simulink model "M46D"  (R2015a)
settings: Solver=ode45  StartTime=0.0  StopTime=20.0  RelTol=1e-4
values from neighbouring files (symbols this model uses):
  d1 = 500    [DePascali4Minit.m]    (also in M46Dinit.m)
  d2 = 500    [DePascali4Minit.m]    (also in M46Dinit.m)
  d3 = 500    [DePascali4Minit.m]    (also in M46Dinit.m)
  d4 = 500    [DePascali4Minit.m]    (also in M46Dinit.m)
  delta1 = 200    [DePascali4Minit.m]    (also in M46Dinit.m)
  delta2 = 200    [DePascali4Minit.m]    (also in M46Dinit.m)
  delta3 = 200    [DePascali4Minit.m]    (also in M46Dinit.m)
  delta4 = 200    [DePascali4Minit.m]    (also in M46Dinit.m)
  g = [0;0;9.81]    [DePascali4Minit.m]    (also in M46Dinit.m)
  j0 = 0.5    [DePascali4Minit.m]    (also in M46Dinit.m)
  j1 = 10    [DePascali4Minit.m]    (also in M46Dinit.m = 1)
  j2 = 10    [DePascali4Minit.m]    (also in M46Dinit.m = 1)
  j3 = 10    [DePascali4Minit.m]    (also in M46Dinit.m = 1)
  j4 = 10    [DePascali4Minit.m]    (also in M46Dinit.m = 1)
  k1 = 50    [DePascali4Minit.m]    (also in M46Dinit.m = 100)
  k2 = 50    [DePascali4Minit.m]    (also in M46Dinit.m = 100)
  k3 = 50    [DePascali4Minit.m]    (also in M46Dinit.m = 100)
  k4 = 50    [DePascali4Minit.m]    (also in M46Dinit.m = 100)
  kappa1 = 10    [DePascali4Minit.m]    (also in M46Dinit.m = 100)
  kappa2 = 10    [DePascali4Minit.m]    (also in M46Dinit.m = 100)
  kappa3 = 10    [DePascali4Minit.m]    (also in M46Dinit.m = 100)
  kappa4 = 10    [DePascali4Minit.m]    (also in M46Dinit.m = 100)
  m0 = 20    [DePascali4Minit.m]    (also in M46Dinit.m)
  m1 = 100    [DePascali4Minit.m]    (also in M46Dinit.m = 10)
  m2 = 100    [DePascali4Minit.m]    (also in M46Dinit.m = 10)
  m3 = 100    [DePascali4Minit.m]    (also in M46Dinit.m = 10)
  m4 = 100    [DePascali4Minit.m]    (also in M46Dinit.m = 10)
  r = [1; 0; 0 ... (first row only)    [DePascali4Minit.m]    (also in M46Dinit.m)
undefined symbols (not defined in the file or in its folder): A, G_Mplus
libraries: aerolibutil x10, aerolibtransform2 x8, dspinverses x3
settings Model: CovSFcnEnable=off  Creator=Martin  LastModifiedBy=mangerer
settings DebuggingCC: SolverPrmCheckMsg=warning

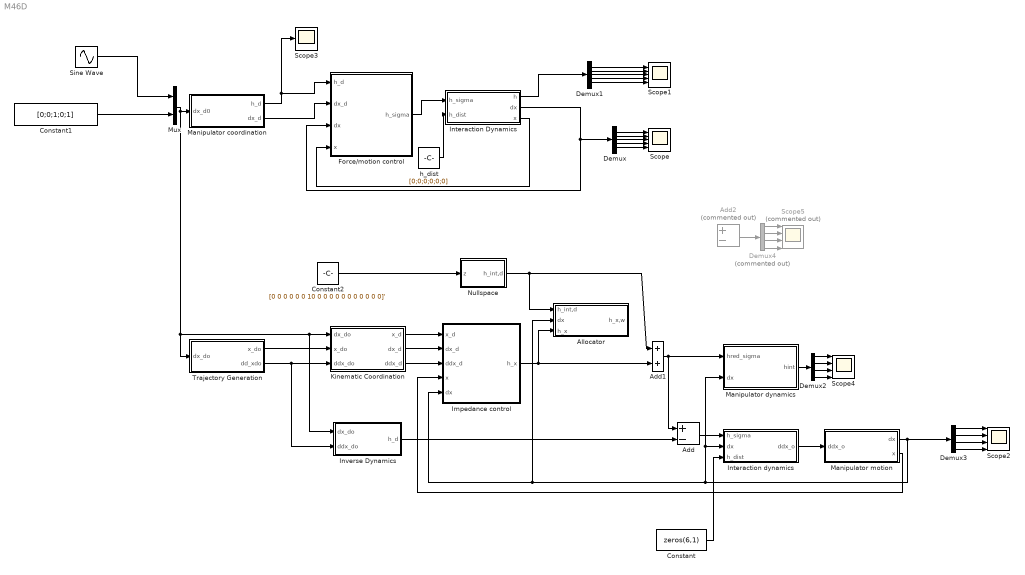
== system M46D ==
  Add : Sum  Inputs=+-
  Add1 : Sum
  Add2 : Sum  Commented=on  Inputs=+-
  Allocator : Subsystem
  Constant : Constant  Value=zeros(6,1)
  Constant1 : Constant  Value=[0;0;1;0;1]
  Constant2 : Constant  Value=[0 0 0 0 0 0 10 0 0 0 0 0 0 0 0 0 0 0]'
  Demux : Demux  Outputs=5
  Demux1 : Demux  Outputs=5
  Demux2 : Demux
  Demux3 : Demux
  Demux4 : Demux  Commented=on
  Force/motion control : Subsystem
  Impedance control : Subsystem
  Interaction Dynamics : Subsystem
  Interaction dynamics : Subsystem
  Inverse Dynamics : Subsystem
  Kinematic Coordination : Subsystem
  Manipulator coordination : Subsystem
  Manipulator dynamics : Subsystem
  Manipulator motion : Subsystem
  Mux : Mux  Inputs=2
  Nullspace : Subsystem
  Scope : Scope  NumInputPorts=5
      settings: ShowLegends=on  YMin=-1.25~-1.25~-2.5~-1.25~-1.5  YMax=1.25~1.25~1.5~1.25~2
  Scope1 : Scope  NumInputPorts=5
      settings: ShowLegends=on  YMin=-50~-100~-100~-5~-5  YMax=200~20~20~5~5
  Scope2 : Scope  NumInputPorts=4
      settings: ShowLegends=on  YMin=-1.25~-2.25~-1.25~-1  YMax=1.25~1.25~1.25~2.25  SaveName=ScopeData2
  Scope3 : Scope
      settings: SaveName=ScopeData5
  Scope4 : Scope  NumInputPorts=4
      settings: ShowLegends=on  YMin=-25~-12.5~-20~-12.5  YMax=20~10~25~7.5  SaveName=ScopeData8
  Scope5 : Scope  Commented=on  NumInputPorts=4
      settings: ShowLegends=on  YMin=-3~-0.5~-0.5~-2.5  YMax=5~2.5~2.5~0.5  SaveName=ScopeData10
  Sine Wave : Sin  SampleTime=0
  Trajectory Generation : Subsystem
  h_dist : Constant  Value=[0;0;0;0;0;0]
  wires:
  Interaction Dynamics/2(dx) -> Force/motion control/3(dx), Demux/1
  Demux/1 -> Scope/1
  Demux/2 -> Scope/2
  Demux/3 -> Scope/3
  Force/motion control/1(h_sigma) -> Interaction Dynamics/1(h_sigma)
  Manipulator coordination/2(dx_d) -> Force/motion control/2(dx_d)
  Interaction Dynamics/1(h) -> Demux1/1
  Demux1/1 -> Scope1/1
  Demux1/2 -> Scope1/2
  Demux1/3 -> Scope1/3
  h_dist/1 -> Interaction Dynamics/2(h_dist)
  Manipulator coordination/1(h_d) -> Force/motion control/1(h_d), Scope3/1
  Mux/1 -> Inverse Dynamics/1(dx_do), Kinematic Coordination/1(dx_do), Trajectory Generation/1(dx_do), Manipulator coordination/1(dx_d0)
  Interaction Dynamics/3(x) -> Force/motion control/4(x)
  Demux1/4 -> Scope1/4
  Demux1/5 -> Scope1/5
  Demux/4 -> Scope/4
  Demux/5 -> Scope/5
  Trajectory Generation/1(x_do) -> Kinematic Coordination/2(x_do)
  Trajectory Generation/2(dd_xdo) -> Inverse Dynamics/2(ddx_do), Kinematic Coordination/3(ddx_do)
  Kinematic Coordination/1(x_d) -> Impedance control/1(x_d)
  Kinematic Coordination/2(dx_d) -> Impedance control/2(dx_d)
  Kinematic Coordination/3(ddx_d) -> Impedance control/3(ddx_d)
  Interaction dynamics/1(ddx_o) -> Manipulator motion/1(ddx_o)
  Impedance control/1(h_x) -> Add1/2, Allocator/3(h_x)
  Inverse Dynamics/1(h_d) -> Add/2
  Add/1 -> Interaction dynamics/1(h_sigma)
  Manipulator motion/1(dx) -> Demux3/1, Allocator/2(dx), Impedance control/5(dx), Interaction dynamics/2(dx), Manipulator dynamics/2(dx)
  Manipulator motion/2(x) -> Impedance control/4(x)
  Constant/1 -> Interaction dynamics/3(h_dist)
  Manipulator dynamics/1(hint) -> Demux2/1
  Demux2/1 -> Scope4/1
  Demux2/2 -> Scope4/2
  Demux2/3 -> Scope4/3
  Demux2/4 -> Scope4/4
  Constant1/1 -> Mux/2
  Sine Wave/1 -> Mux/1
  Demux3/1 -> Scope2/1
  Demux3/2 -> Scope2/2
  Demux3/3 -> Scope2/3
  Demux3/4 -> Scope2/4
  Add1/1 -> Add/1, Manipulator dynamics/1(hred_sigma)
  Constant2/1 -> Nullspace/1(z)
  Demux4/1 -> Scope5/1
  Demux4/2 -> Scope5/2
  Demux4/3 -> Scope5/3
  Demux4/4 -> Scope5/4
  Add2/1 -> Demux4/1
  Nullspace/1(h_int,d) -> Allocator/1(h_int,d), Add1/1

== system M46D/Allocator ==
  h_int,d : Inport
  dx : Inport  Port=2
  h_x : Inport  Port=3
  Add : Sum  Inputs=-+
  Add1 : Sum
  Divide : Product  Inputs=*/*  Multiplication=Matrix(*)
  Divide1 : Product  Inputs=*/*  Multiplication=Matrix(*)
  Divide2 : Product  Inputs=*/*  Multiplication=Matrix(*)
  Inertia : Constant  Value=blkdiag(m1*eye(3), j1*eye(3), m2*eye(3), j2*eye(3), m3*eye(3), j3*eye(3), m4*eye(3), j3*eye(3))
  MATLAB Function : MATLAB Function  TreatAsAtomicUnit=on
  MATLAB Function1 : MATLAB Function  TreatAsAtomicUnit=on
  Math Function : Math  Operator=transpose  SaturateOnIntegerOverflow=on
  h_x,w : Outport
  wires:
  dx/1 -> MATLAB Function1/1(dx)
  Divide/1 -> h_x,w/1
  Math Function/1 -> Divide1/3, Divide/1
  MATLAB Function/1(Ared) -> Math Function/1, Divide2/1, Divide1/1
  Divide1/1 -> Divide/2
  Inertia/1 -> Divide1/2, Divide2/2
  MATLAB Function1/1(bred) -> Add/2
  Add/1 -> Divide/3
  Divide2/1 -> Add/1
  Add1/1 -> Divide2/3
  h_int,d/1 -> Add1/1
  h_x/1 -> Add1/2

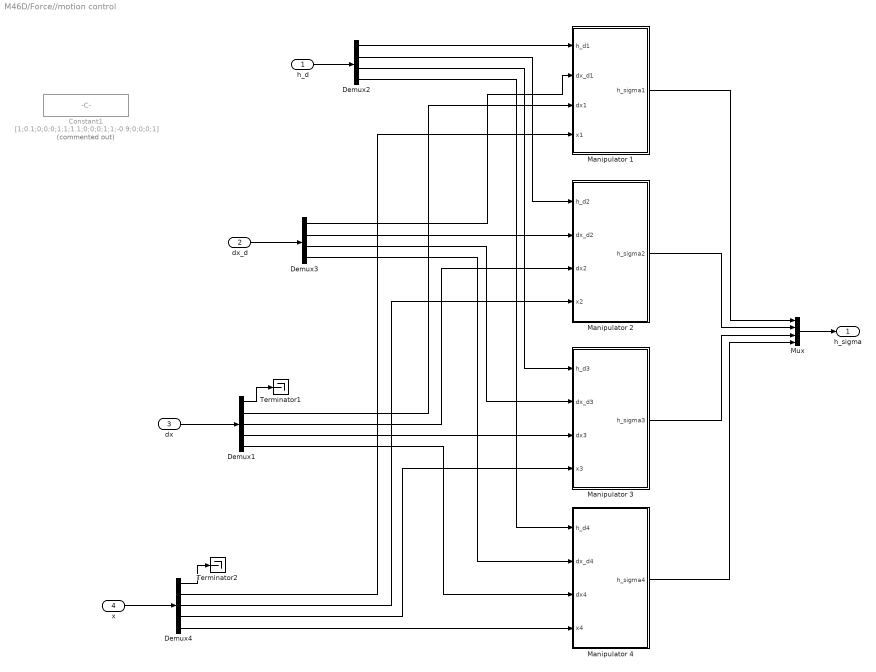
== system M46D/Force//motion control ==
  h_d : Inport
  dx_d : Inport  Port=2
  dx : Inport  Port=3
  x : Inport  Port=4
  Constant1 : Constant  Commented=on  Value=[1;0.1;0;0;0;1;1;1.1;0;0;0;1;1;-0.9;0;0;0;1]
  Demux1 : Demux  Outputs=5
  Demux2 : Demux
  Demux3 : Demux
  Demux4 : Demux  Outputs=5
  Manipulator 1 : Subsystem
  Manipulator 2 : Subsystem
  Manipulator 3 : Subsystem
  Manipulator 4 : Subsystem
  Mux : Mux
  Terminator1 : Terminator
  Terminator2 : Terminator
  h_sigma : Outport
  wires:
  Manipulator 1/1(h_sigma1) -> Mux/1
  Manipulator 2/1(h_sigma2) -> Mux/2
  Mux/1 -> h_sigma/1
  Demux1/1 -> Terminator1/1
  dx_d/1 -> Demux3/1
  h_d/1 -> Demux2/1
  dx/1 -> Demux1/1
  x/1 -> Demux4/1
  Demux4/1 -> Terminator2/1
  Manipulator 3/1(h_sigma3) -> Mux/3
  Manipulator 4/1(h_sigma4) -> Mux/4
  Demux4/5 -> Manipulator 4/4(x4)
  Demux2/1 -> Manipulator 1/1(h_d1)
  Demux2/2 -> Manipulator 2/1(h_d2)
  Demux2/3 -> Manipulator 3/1(h_d3)
  Demux2/4 -> Manipulator 4/1(h_d4)
  Demux3/1 -> Manipulator 1/2(dx_d1)
  Demux3/2 -> Manipulator 2/2(dx_d2)
  Demux3/3 -> Manipulator 3/2(dx_d3)
  Demux3/4 -> Manipulator 4/2(dx_d4)
  Demux1/2 -> Manipulator 1/3(dx1)
  Demux1/3 -> Manipulator 2/3(dx2)
  Demux1/4 -> Manipulator 3/3(dx3)
  Demux1/5 -> Manipulator 4/3(dx4)
  Demux4/4 -> Manipulator 3/4(x3)
  Demux4/3 -> Manipulator 2/4(x2)
  Demux4/2 -> Manipulator 1/4(x1)

== system M46D/Impedance control ==
  x_d : Inport
  dx_d : Inport  Port=2
  ddx_d : Inport  Port=3
  x : Inport  Port=4
  dx : Inport  Port=5
  Demux{,1..4} (5 alike) : Demux
  Manipulator1 : Subsystem
  Manipulator2 : Subsystem
  Manipulator3 : Subsystem
  Manipulator4 : Subsystem
  Mux : Mux
  h_x : Outport
  wires:
  dx/1 -> Demux4/1
  x/1 -> Demux3/1
  ddx_d/1 -> Demux2/1
  dx_d/1 -> Demux1/1
  x_d/1 -> Demux/1
  Demux/1 -> Manipulator1/1(x_d1)
  Demux/2 -> Manipulator2/1(x_d2)
  Demux/3 -> Manipulator3/1(x_d3)
  Demux/4 -> Manipulator4/1(x_d4)
  Demux1/1 -> Manipulator1/2(dx_d1)
  Demux1/2 -> Manipulator2/2(dx_d2)
  Demux1/3 -> Manipulator3/2(dx_d3)
  Demux1/4 -> Manipulator4/2(dx_d4)
  Demux2/1 -> Manipulator1/3(ddx_d1)
  Demux2/2 -> Manipulator2/3(ddx_d2)
  Demux2/3 -> Manipulator3/3(ddx_d3)
  Demux2/4 -> Manipulator4/3(ddx_d4)
  Demux3/1 -> Manipulator1/4(x1)
  Demux3/2 -> Manipulator2/4(x2)
  Demux3/3 -> Manipulator3/4(x3)
  Demux3/4 -> Manipulator4/4(x4)
  Demux4/4 -> Manipulator4/5(dx4)
  Demux4/3 -> Manipulator3/5(dx3)
  Demux4/2 -> Manipulator2/5(dx2)
  Demux4/1 -> Manipulator1/5(dx1)
  Mux/1 -> h_x/1
  Manipulator1/1(h_x1) -> Mux/1
  Manipulator2/1(h_x2) -> Mux/2
  Manipulator3/1(h_x3) -> Mux/3
  Manipulator4/1(h_x4) -> Mux/4

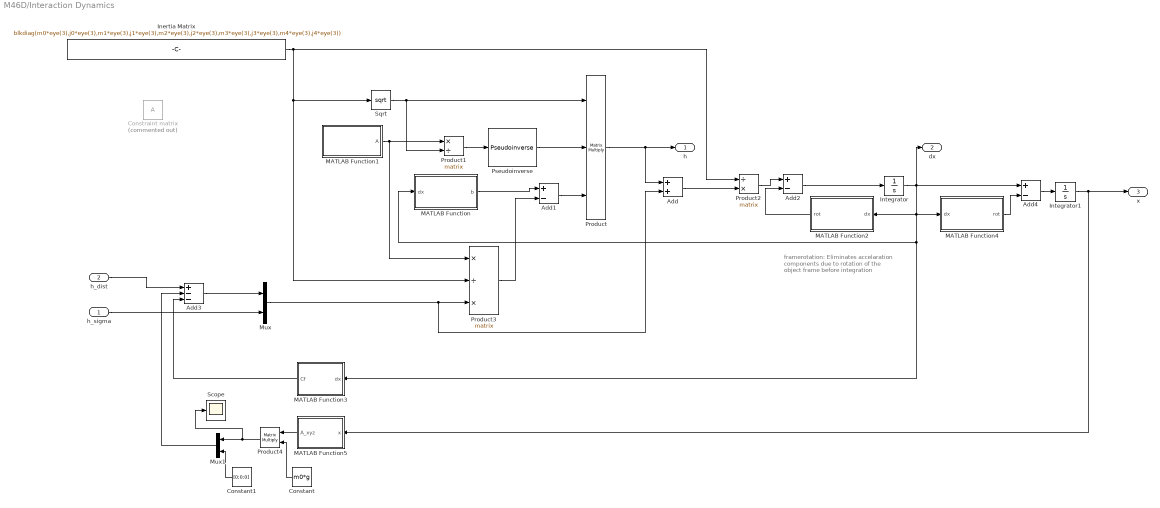
== system M46D/Interaction Dynamics ==
  note: framerotation: Eliminates accelaration
      |  components  due to rotation of the
      |  object frame before integration
  h_sigma : Inport
  h_dist : Inport  Port=2
  Add : Sum
  Add1 : Sum  Inputs=+-
  Add2 : Sum  Inputs=+-
  Add3 : Sum  Inputs=+--
  Add4 : Sum  Inputs=+-
  Constant : Constant  Value=m0*g
  Constant1 : Constant  Value=[0;0;0]
  Constraint matrix : Constant  Commented=on  Value=A
  Inertia Matrix : Constant  Value=blkdiag(m0*eye(3),j0*eye(3),m1*eye(3),j1*eye(3),m2*eye(3),j2*eye(3),m3*eye(3),j3*eye(3),m4*eye(3),j4*eye(3))
  Integrator : Integrator
  Integrator1 : Integrator
  MATLAB Function : MATLAB Function  TreatAsAtomicUnit=on
  MATLAB Function1 : MATLAB Function  TreatAsAtomicUnit=on
  MATLAB Function2 : MATLAB Function  TreatAsAtomicUnit=on
  MATLAB Function3 : MATLAB Function  TreatAsAtomicUnit=on
  MATLAB Function4 : MATLAB Function  TreatAsAtomicUnit=on
  MATLAB Function5 : MATLAB Function  TreatAsAtomicUnit=on
  Mux : Mux  Inputs=2
  Mux1 : Mux  Inputs=2
  Product : Product  Inputs=***  Multiplication=Matrix(*)
  Product1 : Product  Inputs=*/  Multiplication=Matrix(*)
  Product2 : Product  Inputs=/*  Multiplication=Matrix(*)
  Product3 : Product  Inputs=*/*  Multiplication=Matrix(*)
  Product4 : Product  Multiplication=Matrix(*)
  Pseudoinverse : dspinverses/Pseudoinverse  wanterr=off
  Scope : Scope
      settings: ShowLegends=on  SaveName=ScopeData6
  Sqrt : Sqrt  SaturateOnIntegerOverflow=on
  h : Outport
  dx : Outport  Port=2
  x : Outport  Port=3
  wires:
  Sqrt/1 -> Product/1, Product1/2
  Pseudoinverse/1 -> Product/2
  Product1/1 -> Pseudoinverse/1
  Integrator/1 -> dx/1, Add4/1, MATLAB Function4/1(dx), MATLAB Function2/1(dx), MATLAB Function3/1(dx), MATLAB Function/1(dx)
  Product/1 -> h/1, Add/1
  Add/1 -> Product2/2
  Inertia Matrix/1 -> Product2/1, Sqrt/1, Product3/2
  h_sigma/1 -> Mux/2
  Add1/1 -> Product/3
  MATLAB Function/1(b) -> Add1/1
  Product3/1 -> Add1/2
  Mux/1 -> Add/2, Product3/3
  MATLAB Function1/1(A) -> Product1/1, Product3/1
  Product2/1 -> Add2/1
  Add2/1 -> Integrator/1
  MATLAB Function2/1(rot) -> Add2/2
  Add3/1 -> Mux/1
  h_dist/1 -> Add3/1
  Integrator1/1 -> MATLAB Function5/1(x), x/1
  Add4/1 -> Integrator1/1
  MATLAB Function4/1(rot) -> Add4/2
  MATLAB Function5/1(A_xyz) -> Product4/1
  MATLAB Function3/1(Cf) -> Add3/3
  Constant/1 -> Product4/2
  Product4/1 -> Scope/1, Mux1/1
  Constant1/1 -> Mux1/2
  Mux1/1 -> Add3/2

== system M46D/Interaction dynamics ==
  h_sigma : Inport
  dx : Inport  Port=2
  h_dist : Inport  Port=3
  Add : Sum  Inputs=++-
  Add1 : Sum  Inputs=+--
  Gravitation : Constant  Value=[-m0*g;zeros(3,1)]
  Inertia : Constant  Value=blkdiag(m1*eye(3), j1*eye(3), m2*eye(3), j2*eye(3), m3*eye(3), j3*eye(3), m4*eye(3), j3*eye(3))
  MATLAB Function : MATLAB Function  TreatAsAtomicUnit=on
  MATLAB Function1 : MATLAB Function  TreatAsAtomicUnit=on
  MATLAB Function2 : MATLAB Function  TreatAsAtomicUnit=on
  MATLAB Function3 : MATLAB Function  TreatAsAtomicUnit=on
  Product : Product  Inputs=/*  Multiplication=Matrix(*)
  Product1 : Product  Multiplication=Matrix(*)
  Product3 : Product  Inputs=***  Multiplication=Matrix(*)
  ddx_o : Outport
  wires:
  MATLAB Function3/1(G) -> Product1/1, Product3/1, MATLAB Function/1(G)
  Inertia/1 -> Product3/2, MATLAB Function/2(M)
  MATLAB Function/1(Mapp) -> Product/1
  Add/1 -> Product/2
  Product1/1 -> Add/2
  h_sigma/1 -> Product1/2
  Add1/1 -> Add/1
  h_dist/1 -> Add1/1
  Gravitation/1 -> Add1/2
  dx/1 -> MATLAB Function2/1(dx), MATLAB Function1/1(dx)
  MATLAB Function1/1(hcoriolis) -> Add1/3
  Product3/1 -> Add/3
  MATLAB Function2/1(b) -> Product3/3
  Product/1 -> ddx_o/1

== system M46D/Inverse Dynamics ==
  dx_do : Inport
  ddx_do : Inport  Port=2
  Add : Sum  Inputs=+++
  Gravitation : Constant  Value=[-m0*g;zeros(3,1)]
  MATLAB Function : MATLAB Function  TreatAsAtomicUnit=on
  MATLAB Function3 : MATLAB Function  TreatAsAtomicUnit=on
  Object Inertia : Constant  Value=blkdiag(m0*eye(3),j0*eye(3));
  Product : Product  Multiplication=Matrix(*)
  Product1 : Product  Multiplication=Matrix(*)
  Product2 : Product  Multiplication=Matrix(*)
  Pseudoinverse : dspinverses/Pseudoinverse  wanterr=off
  h_d : Outport
  wires:
  ddx_do/1 -> Product/2
  Object Inertia/1 -> Product/1
  Product/1 -> Add/3
  dx_do/1 -> Product1/2, MATLAB Function/1(dx_do)
  MATLAB Function/1(C_o) -> Product1/1
  Product1/1 -> Add/2
  Gravitation/1 -> Add/1
  MATLAB Function3/1(G) -> Pseudoinverse/1
  Add/1 -> Product2/2
  Pseudoinverse/1 -> Product2/1
  Product2/1 -> h_d/1

== system M46D/Kinematic Coordination ==
  dx_do : Inport
  x_do : Inport  Port=2
  ddx_do : Inport  Port=3
  Add : Sum
  Demux : Demux  Outputs=7
  MATLAB Function : MATLAB Function  TreatAsAtomicUnit=on
  MATLAB Function1 : MATLAB Function  TreatAsAtomicUnit=on
  MATLAB Function3 : MATLAB Function  TreatAsAtomicUnit=on
  Math Function : Math  Operator=transpose  SaturateOnIntegerOverflow=on
  Mux : Mux  Inputs=3
  Mux1 : Mux
  Product : Product  Multiplication=Matrix(*)
  Product1 : Product  Multiplication=Matrix(*)
  x_d : Outport
  dx_d : Outport  Port=2
  ddx_d : Outport  Port=3
  wires:
  MATLAB Function3/1(G) -> Math Function/1
  Math Function/1 -> Product1/1, Product/1
  dx_do/1 -> MATLAB Function1/1(dx_do), Product/2
  Product/1 -> dx_d/1
  x_do/1 -> Demux/1
  Demux/1 -> Mux/1
  Demux/2 -> Mux/2
  Demux/3 -> Mux/3
  Demux/5 -> Mux1/2
  Demux/6 -> Mux1/3
  Demux/7 -> Mux1/4
  Demux/4 -> Mux1/1
  Mux1/1 -> MATLAB Function/2(q_do)
  Mux/1 -> MATLAB Function/1(p_do)
  MATLAB Function/1(x_d) -> x_d/1
  MATLAB Function1/1(b) -> Add/1
  ddx_do/1 -> Product1/2
  Product1/1 -> Add/2
  Add/1 -> ddx_d/1

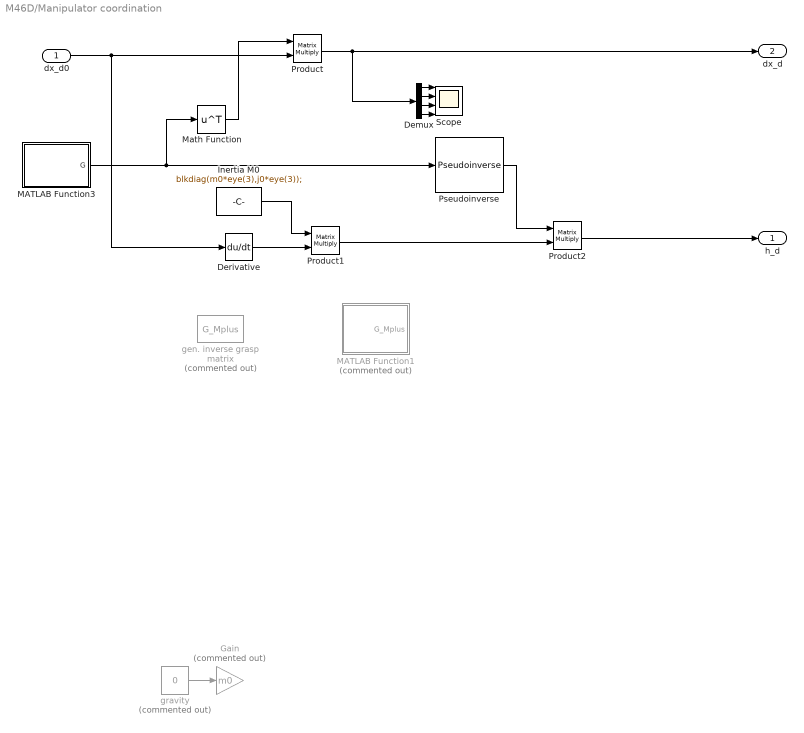
== system M46D/Manipulator coordination ==
  dx_d0 : Inport
  Demux : Demux
  Derivative : Derivative
  Gain : Gain  Commented=on  Gain=m0
  Inertia M0 : Constant  Value=blkdiag(m0*eye(3),j0*eye(3));
  MATLAB Function1 : MATLAB Function  Commented=on  TreatAsAtomicUnit=on
  MATLAB Function3 : MATLAB Function  TreatAsAtomicUnit=on
  Math Function : Math  Operator=transpose  SaturateOnIntegerOverflow=on
  Product : Product  Multiplication=Matrix(*)
  Product1 : Product  Multiplication=Matrix(*)
  Product2 : Product  Multiplication=Matrix(*)
  Pseudoinverse : dspinverses/Pseudoinverse  wanterr=off
  Scope : Scope  NumInputPorts=4
      settings: ShowLegends=on  YMin=-5~-5~-5~-5  YMax=5~5~5~5  SaveName=ScopeData3
  gen. inverse grasp matrix : Constant  Commented=on  Value=G_Mplus
  gravity : Constant  Commented=on  Value=0
  h_d : Outport
  dx_d : Outport  Port=2
  wires:
  dx_d0/1 -> Product/2, Derivative/1
  Math Function/1 -> Product/1
  Product/1 -> Demux/1, dx_d/1
  Derivative/1 -> Product1/2
  gravity/1 -> Gain/1
  Product1/1 -> Product2/2
  Product2/1 -> h_d/1
  Demux/1 -> Scope/1
  Demux/2 -> Scope/2
  Demux/3 -> Scope/3
  Demux/4 -> Scope/4
  Inertia M0/1 -> Product1/1
  MATLAB Function3/1(G) -> Pseudoinverse/1, Math Function/1
  Pseudoinverse/1 -> Product2/1

== system M46D/Manipulator dynamics ==
  hred_sigma : Inport
  dx : Inport  Port=2
  Add : Sum  Inputs=-+
  Divide : Product  Inputs=*/*  Multiplication=Matrix(*)
  Divide1 : Product  Inputs=*/*  Multiplication=Matrix(*)
  Divide2 : Product  Inputs=*/*  Multiplication=Matrix(*)
  Inertia : Constant  Value=blkdiag(m1*eye(3), j1*eye(3), m2*eye(3), j2*eye(3), m3*eye(3), j3*eye(3), m4*eye(3), j3*eye(3))
  MATLAB Function : MATLAB Function  TreatAsAtomicUnit=on
  MATLAB Function1 : MATLAB Function  TreatAsAtomicUnit=on
  Math Function : Math  Operator=transpose  SaturateOnIntegerOverflow=on
  hint : Outport
  wires:
  Divide/1 -> hint/1
  Math Function/1 -> Divide1/3, Divide/1
  MATLAB Function/1(Ared) -> Math Function/1, Divide2/1, Divide1/1
  Divide1/1 -> Divide/2
  Inertia/1 -> Divide1/2, Divide2/2
  dx/1 -> MATLAB Function1/1(dx)
  MATLAB Function1/1(bred) -> Add/2
  Add/1 -> Divide/3
  Divide2/1 -> Add/1
  hred_sigma/1 -> Divide2/3

== system M46D/Manipulator motion ==
  ddx_o : Inport
  AngVelo2Quat : Subsystem
  Demux : Demux  Outputs=2
  Integrator : Integrator  InitialCondition=zeros(6,1)
  Integrator1 : Integrator  InitialCondition=[0 0 0]'
  MATLAB Function : MATLAB Function  TreatAsAtomicUnit=on
  MATLAB Function3 : MATLAB Function  TreatAsAtomicUnit=on
  Math Function : Math  Operator=transpose  SaturateOnIntegerOverflow=on
  Product : Product  Multiplication=Matrix(*)
  dx : Outport
  x : Outport  Port=2
  wires:
  ddx_o/1 -> Integrator/1
  Integrator/1 -> Product/2, Demux/1
  MATLAB Function3/1(G) -> Math Function/1
  Math Function/1 -> Product/1
  Product/1 -> dx/1
  Demux/2 -> AngVelo2Quat/1(omega_o)
  Demux/1 -> Integrator1/1
  AngVelo2Quat/1(q_o) -> MATLAB Function/2(q_o)
  Integrator1/1 -> MATLAB Function/1(p_o)
  MATLAB Function/1(x) -> x/1

== system M46D/Nullspace ==
  z : Inport
  MATLAB Function : MATLAB Function  TreatAsAtomicUnit=on
  Math Function : Math  Operator=transpose  SaturateOnIntegerOverflow=on
  Product : Product  Multiplication=Matrix(*)
  h_int,d : Outport
  wires:
  MATLAB Function/1(Ared) -> Math Function/1
  Math Function/1 -> Product/1
  z/1 -> Product/2
  Product/1 -> h_int,d/1

== system M46D/Trajectory Generation ==
  dx_do : Inport
  AngVelo2Quat : Subsystem
  Demux : Demux  Outputs=2
  Derivative : Derivative
  Integrator : Integrator
  Mux : Mux  Inputs=2
  x_do : Outport
  dd_xdo : Outport  Port=2
  wires:
  dx_do/1 -> Derivative/1, Demux/1
  Demux/2 -> AngVelo2Quat/1(omega_do)
  Demux/1 -> Integrator/1
  AngVelo2Quat/1(q_do) -> Mux/2
  Integrator/1 -> Mux/1
  Mux/1 -> x_do/1
  Derivative/1 -> dd_xdo/1

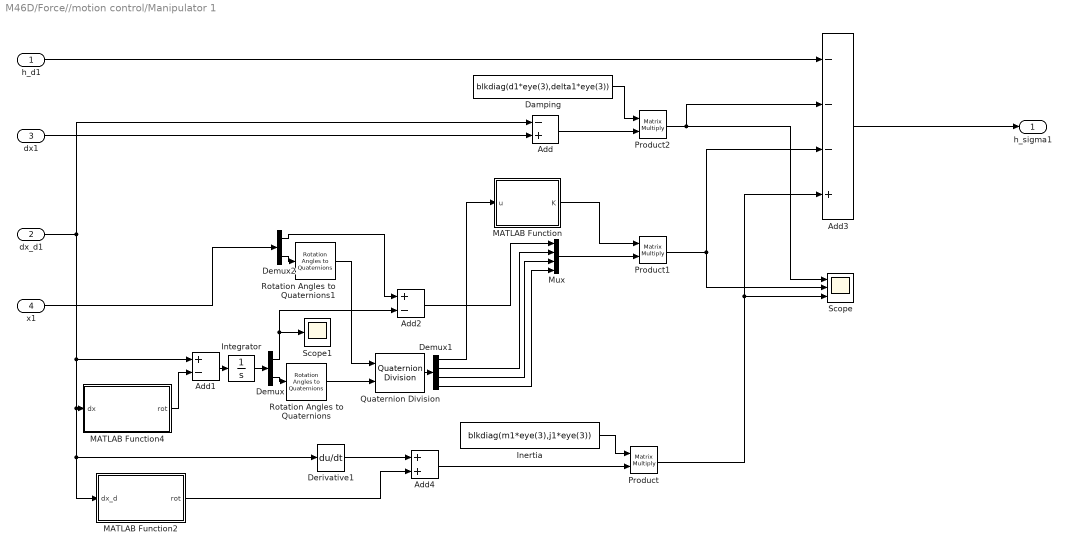
== system M46D/Force//motion control/Manipulator 1 ==
  h_d1 : Inport
  dx_d1 : Inport  Port=2
  dx1 : Inport  Port=3
  x1 : Inport  Port=4
  Add : Sum  Inputs=-+
  Add1 : Sum  Inputs=+-
  Add2 : Sum  Inputs=+-
  Add3 : Sum  Inputs=---+
  Add4 : Sum
  Damping : Constant  Value=blkdiag(d1*eye(3),delta1*eye(3))
  Demux : Demux  Outputs=2
  Demux1 : Demux
  Demux2 : Demux  Outputs=2
  Derivative1 : Derivative
  Inertia : Constant  Value=blkdiag(m1*eye(3),j1*eye(3))
  Integrator : Integrator
  MATLAB Function : MATLAB Function  TreatAsAtomicUnit=on
  MATLAB Function2 : MATLAB Function  TreatAsAtomicUnit=on
  MATLAB Function4 : MATLAB Function  TreatAsAtomicUnit=on
  Mux : Mux
  Product : Product  Multiplication=Matrix(*)
  Product1 : Product  Multiplication=Matrix(*)
  Product2 : Product  Multiplication=Matrix(*)
  Quaternion Division : aerolibutil/Quaternion Division
  Rotation Angles to Quaternions : aerolibtransform2/Rotation Angles to Quaternions  rotationOrder=XYZ
  Rotation Angles to Quaternions1 : aerolibtransform2/Rotation Angles to Quaternions  rotationOrder=XYZ
  Scope : Scope  NumInputPorts=3
      settings: ShowLegends=on  YMin=-5~-5~-5  YMax=5~5~5  SaveName=ScopeData4
  Scope1 : Scope
      settings: ShowLegends=on  SaveName=ScopeData7
  h_sigma1 : Outport
  wires:
  dx_d1/1 -> Add1/1, Derivative1/1, MATLAB Function2/1(dx_d), MATLAB Function4/1(dx), Add/1
  Mux/1 -> Product1/2
  Add/1 -> Product2/2
  Damping/1 -> Product2/1
  Inertia/1 -> Product/1
  Product/1 -> Scope/3, Add3/4
  h_d1/1 -> Add3/1
  Add3/1 -> h_sigma1/1
  Integrator/1 -> Demux/1
  Demux/2 -> Rotation Angles to Quaternions/1
  dx1/1 -> Add/2
  x1/1 -> Demux2/1
  Demux2/2 -> Rotation Angles to Quaternions1/1
  MATLAB Function/1(K) -> Product1/1
  Rotation Angles to Quaternions1/1 -> Quaternion Division/1
  Rotation Angles to Quaternions/1 -> Quaternion Division/2
  Quaternion Division/1 -> Demux1/1
  Demux1/1 -> MATLAB Function/1(u)
  Demux2/1 -> Add2/1
  Demux/1 -> Scope1/1, Add2/2
  Add2/1 -> Mux/1
  Demux1/2 -> Mux/2
  Demux1/3 -> Mux/3
  Demux1/4 -> Mux/4
  Product2/1 -> Scope/1, Add3/2
  Product1/1 -> Add3/3, Scope/2
  MATLAB Function4/1(rot) -> Add1/2
  Add1/1 -> Integrator/1
  Add4/1 -> Product/2
  Derivative1/1 -> Add4/1
  MATLAB Function2/1(rot) -> Add4/2

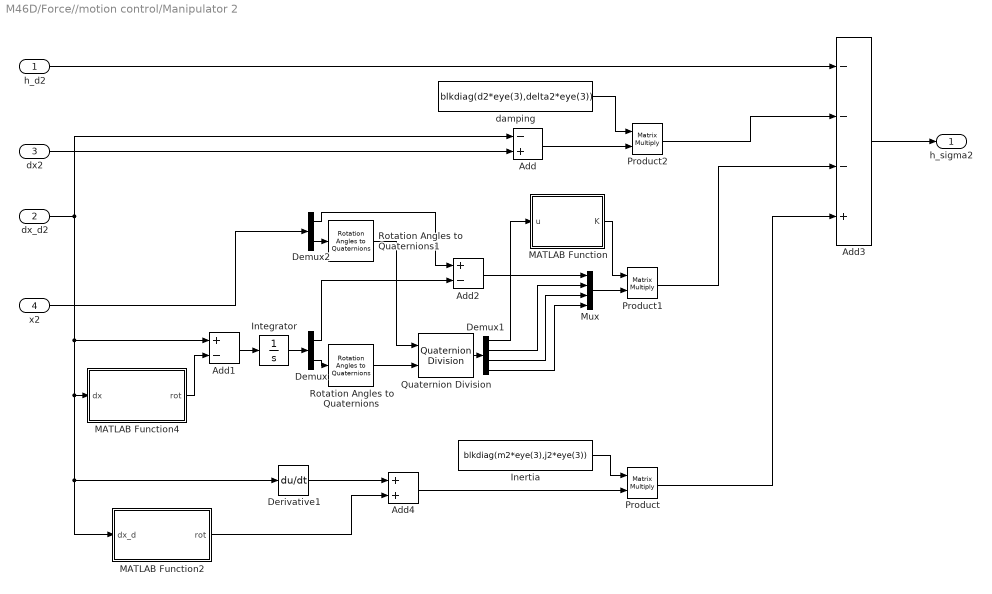
== system M46D/Force//motion control/Manipulator 2 ==
  h_d2 : Inport
  dx_d2 : Inport  Port=2
  dx2 : Inport  Port=3
  x2 : Inport  Port=4
  Add : Sum  Inputs=-+
  Add1 : Sum  Inputs=+-
  Add2 : Sum  Inputs=+-
  Add3 : Sum  Inputs=---+
  Add4 : Sum
  Demux : Demux  Outputs=2
  Demux1 : Demux
  Demux2 : Demux  Outputs=2
  Derivative1 : Derivative
  Inertia : Constant  Value=blkdiag(m2*eye(3),j2*eye(3))
  Integrator : Integrator
  MATLAB Function : MATLAB Function  TreatAsAtomicUnit=on
  MATLAB Function2 : MATLAB Function  TreatAsAtomicUnit=on
  MATLAB Function4 : MATLAB Function  TreatAsAtomicUnit=on
  Mux : Mux
  Product : Product  Multiplication=Matrix(*)
  Product1 : Product  Multiplication=Matrix(*)
  Product2 : Product  Multiplication=Matrix(*)
  Quaternion Division : aerolibutil/Quaternion Division
  Rotation Angles to Quaternions : aerolibtransform2/Rotation Angles to Quaternions  rotationOrder=XYZ
  Rotation Angles to Quaternions1 : aerolibtransform2/Rotation Angles to Quaternions  rotationOrder=XYZ
  damping : Constant  Value=blkdiag(d2*eye(3),delta2*eye(3))
  h_sigma2 : Outport
  wires:
  dx_d2/1 -> Add/1, Add1/1, Derivative1/1, MATLAB Function2/1(dx_d), MATLAB Function4/1(dx)
  dx2/1 -> Add/2
  Add/1 -> Product2/2
  damping/1 -> Product2/1
  Inertia/1 -> Product/1
  Product/1 -> Add3/4
  h_d2/1 -> Add3/1
  Add3/1 -> h_sigma2/1
  Integrator/1 -> Demux/1
  Demux/2 -> Rotation Angles to Quaternions/1
  x2/1 -> Demux2/1
  Demux2/2 -> Rotation Angles to Quaternions1/1
  MATLAB Function/1(K) -> Product1/1
  Mux/1 -> Product1/2
  Rotation Angles to Quaternions/1 -> Quaternion Division/2
  Rotation Angles to Quaternions1/1 -> Quaternion Division/1
  Quaternion Division/1 -> Demux1/1
  Demux1/1 -> MATLAB Function/1(u)
  Add2/1 -> Mux/1
  Demux2/1 -> Add2/1
  Demux/1 -> Add2/2
  Demux1/2 -> Mux/2
  Demux1/3 -> Mux/3
  Demux1/4 -> Mux/4
  Product2/1 -> Add3/2
  Product1/1 -> Add3/3
  Add1/1 -> Integrator/1
  MATLAB Function4/1(rot) -> Add1/2
  MATLAB Function2/1(rot) -> Add4/2
  Add4/1 -> Product/2
  Derivative1/1 -> Add4/1

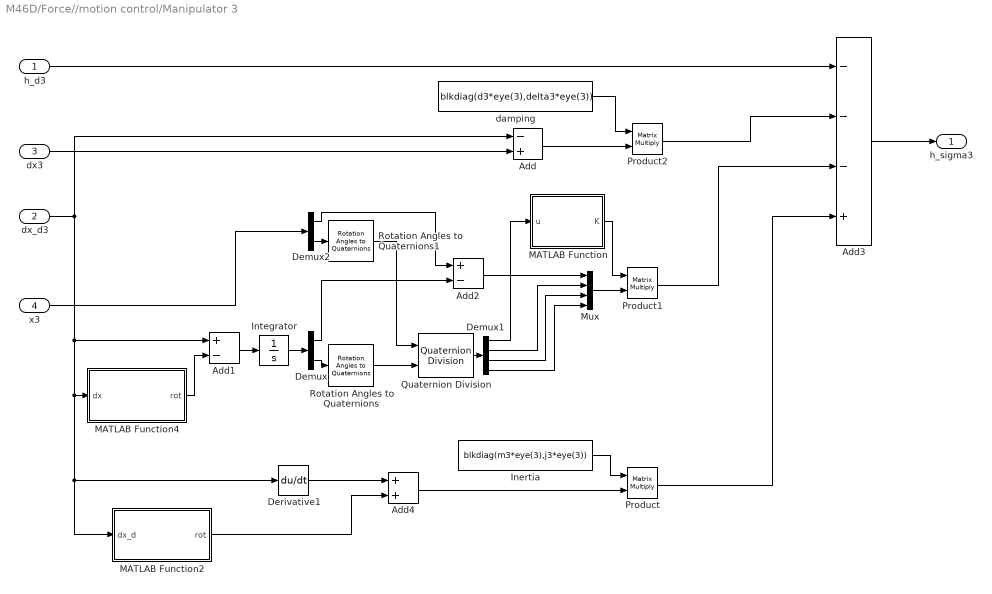
== system M46D/Force//motion control/Manipulator 3 ==
  h_d3 : Inport
  dx_d3 : Inport  Port=2
  dx3 : Inport  Port=3
  x3 : Inport  Port=4
  Add : Sum  Inputs=-+
  Add1 : Sum  Inputs=+-
  Add2 : Sum  Inputs=+-
  Add3 : Sum  Inputs=---+
  Add4 : Sum
  Demux : Demux  Outputs=2
  Demux1 : Demux
  Demux2 : Demux  Outputs=2
  Derivative1 : Derivative
  Inertia : Constant  Value=blkdiag(m3*eye(3),j3*eye(3))
  Integrator : Integrator
  MATLAB Function : MATLAB Function  TreatAsAtomicUnit=on
  MATLAB Function2 : MATLAB Function  TreatAsAtomicUnit=on
  MATLAB Function4 : MATLAB Function  TreatAsAtomicUnit=on
  Mux : Mux
  Product : Product  Multiplication=Matrix(*)
  Product1 : Product  Multiplication=Matrix(*)
  Product2 : Product  Multiplication=Matrix(*)
  Quaternion Division : aerolibutil/Quaternion Division
  Rotation Angles to Quaternions : aerolibtransform2/Rotation Angles to Quaternions  rotationOrder=XYZ
  Rotation Angles to Quaternions1 : aerolibtransform2/Rotation Angles to Quaternions  rotationOrder=XYZ
  damping : Constant  Value=blkdiag(d3*eye(3),delta3*eye(3))
  h_sigma3 : Outport
  wires:
  dx_d3/1 -> Add/1, Add1/1, Derivative1/1, MATLAB Function2/1(dx_d), MATLAB Function4/1(dx)
  dx3/1 -> Add/2
  Add/1 -> Product2/2
  damping/1 -> Product2/1
  Inertia/1 -> Product/1
  Product/1 -> Add3/4
  h_d3/1 -> Add3/1
  Add3/1 -> h_sigma3/1
  Integrator/1 -> Demux/1
  Demux/2 -> Rotation Angles to Quaternions/1
  x3/1 -> Demux2/1
  Demux2/2 -> Rotation Angles to Quaternions1/1
  MATLAB Function/1(K) -> Product1/1
  Mux/1 -> Product1/2
  Rotation Angles to Quaternions/1 -> Quaternion Division/2
  Rotation Angles to Quaternions1/1 -> Quaternion Division/1
  Quaternion Division/1 -> Demux1/1
  Demux1/1 -> MATLAB Function/1(u)
  Add2/1 -> Mux/1
  Demux2/1 -> Add2/1
  Demux/1 -> Add2/2
  Demux1/2 -> Mux/2
  Demux1/3 -> Mux/3
  Demux1/4 -> Mux/4
  Product2/1 -> Add3/2
  Product1/1 -> Add3/3
  Add1/1 -> Integrator/1
  MATLAB Function4/1(rot) -> Add1/2
  MATLAB Function2/1(rot) -> Add4/2
  Add4/1 -> Product/2
  Derivative1/1 -> Add4/1

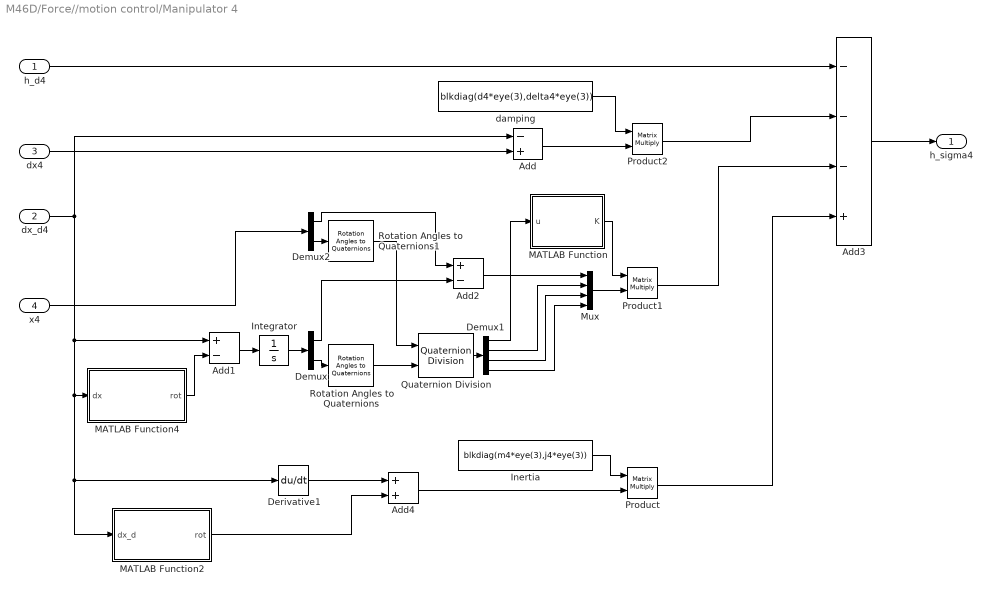
== system M46D/Force//motion control/Manipulator 4 ==
  h_d4 : Inport
  dx_d4 : Inport  Port=2
  dx4 : Inport  Port=3
  x4 : Inport  Port=4
  Add : Sum  Inputs=-+
  Add1 : Sum  Inputs=+-
  Add2 : Sum  Inputs=+-
  Add3 : Sum  Inputs=---+
  Add4 : Sum
  Demux : Demux  Outputs=2
  Demux1 : Demux
  Demux2 : Demux  Outputs=2
  Derivative1 : Derivative
  Inertia : Constant  Value=blkdiag(m4*eye(3),j4*eye(3))
  Integrator : Integrator
  MATLAB Function : MATLAB Function  TreatAsAtomicUnit=on
  MATLAB Function2 : MATLAB Function  TreatAsAtomicUnit=on
  MATLAB Function4 : MATLAB Function  TreatAsAtomicUnit=on
  Mux : Mux
  Product : Product  Multiplication=Matrix(*)
  Product1 : Product  Multiplication=Matrix(*)
  Product2 : Product  Multiplication=Matrix(*)
  Quaternion Division : aerolibutil/Quaternion Division
  Rotation Angles to Quaternions : aerolibtransform2/Rotation Angles to Quaternions  rotationOrder=XYZ
  Rotation Angles to Quaternions1 : aerolibtransform2/Rotation Angles to Quaternions  rotationOrder=XYZ
  damping : Constant  Value=blkdiag(d4*eye(3),delta4*eye(3))
  h_sigma4 : Outport
  wires:
  dx_d4/1 -> Add/1, Add1/1, Derivative1/1, MATLAB Function2/1(dx_d), MATLAB Function4/1(dx)
  dx4/1 -> Add/2
  Add/1 -> Product2/2
  damping/1 -> Product2/1
  Inertia/1 -> Product/1
  Product/1 -> Add3/4
  h_d4/1 -> Add3/1
  Add3/1 -> h_sigma4/1
  Integrator/1 -> Demux/1
  Demux/2 -> Rotation Angles to Quaternions/1
  x4/1 -> Demux2/1
  Demux2/2 -> Rotation Angles to Quaternions1/1
  MATLAB Function/1(K) -> Product1/1
  Mux/1 -> Product1/2
  Rotation Angles to Quaternions/1 -> Quaternion Division/2
  Rotation Angles to Quaternions1/1 -> Quaternion Division/1
  Quaternion Division/1 -> Demux1/1
  Demux1/1 -> MATLAB Function/1(u)
  Add2/1 -> Mux/1
  Demux2/1 -> Add2/1
  Demux/1 -> Add2/2
  Demux1/2 -> Mux/2
  Demux1/3 -> Mux/3
  Demux1/4 -> Mux/4
  Product2/1 -> Add3/2
  Product1/1 -> Add3/3
  Add1/1 -> Integrator/1
  MATLAB Function4/1(rot) -> Add1/2
  MATLAB Function2/1(rot) -> Add4/2
  Add4/1 -> Product/2
  Derivative1/1 -> Add4/1

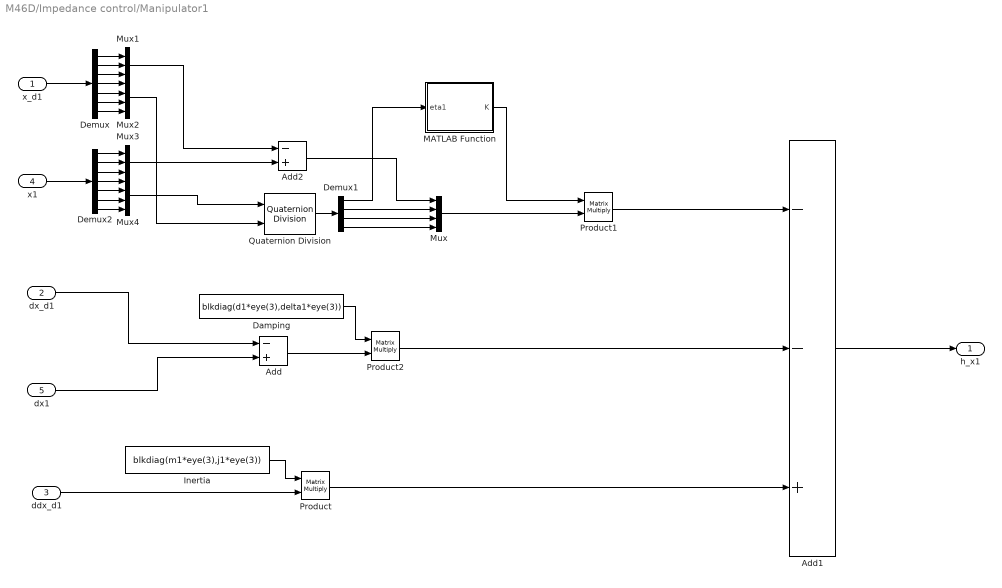
== system M46D/Impedance control/Manipulator1 ==
  x_d1 : Inport
  dx_d1 : Inport  Port=2
  ddx_d1 : Inport  Port=3
  x1 : Inport  Port=4
  dx1 : Inport  Port=5
  Add : Sum  Inputs=-+
  Add1 : Sum  Inputs=--+
  Add2 : Sum  Inputs=-+
  Damping : Constant  Value=blkdiag(d1*eye(3),delta1*eye(3))
  Demux : Demux  Outputs=7
  Demux1 : Demux
  Demux2 : Demux  Outputs=7
  Inertia : Constant  Value=blkdiag(m1*eye(3),j1*eye(3))
  MATLAB Function : MATLAB Function  TreatAsAtomicUnit=on
  Mux : Mux
  Mux1 : Mux  Inputs=3
  Mux2 : Mux
  Mux3 : Mux  Inputs=3
  Mux4 : Mux
  Product : Product  Multiplication=Matrix(*)
  Product1 : Product  Multiplication=Matrix(*)
  Product2 : Product  Multiplication=Matrix(*)
  Quaternion Division : aerolibutil/Quaternion Division
  h_x1 : Outport
  wires:
  Add/1 -> Product2/2
  Damping/1 -> Product2/1
  dx_d1/1 -> Add/1
  dx1/1 -> Add/2
  MATLAB Function/1(K) -> Product1/1
  Demux1/1 -> MATLAB Function/1(eta1)
  Add2/1 -> Mux/1
  Demux1/2 -> Mux/2
  Demux1/3 -> Mux/3
  Demux1/4 -> Mux/4
  x1/1 -> Demux2/1
  x_d1/1 -> Demux/1
  Demux/2 -> Mux1/2
  Demux/1 -> Mux1/1
  Demux/3 -> Mux1/3
  Demux/4 -> Mux2/1
  Demux/5 -> Mux2/2
  Demux/6 -> Mux2/3
  Demux/7 -> Mux2/4
  Demux2/2 -> Mux3/2
  Demux2/1 -> Mux3/1
  Demux2/3 -> Mux3/3
  Demux2/4 -> Mux4/1
  Demux2/5 -> Mux4/2
  Demux2/6 -> Mux4/3
  Demux2/7 -> Mux4/4
  Mux1/1 -> Add2/1
  Mux3/1 -> Add2/2
  Quaternion Division/1 -> Demux1/1
  Mux4/1 -> Quaternion Division/1
  Mux2/1 -> Quaternion Division/2
  Mux/1 -> Product1/2
  Inertia/1 -> Product/1
  ddx_d1/1 -> Product/2
  Add1/1 -> h_x1/1
  Product1/1 -> Add1/1
  Product2/1 -> Add1/2
  Product/1 -> Add1/3

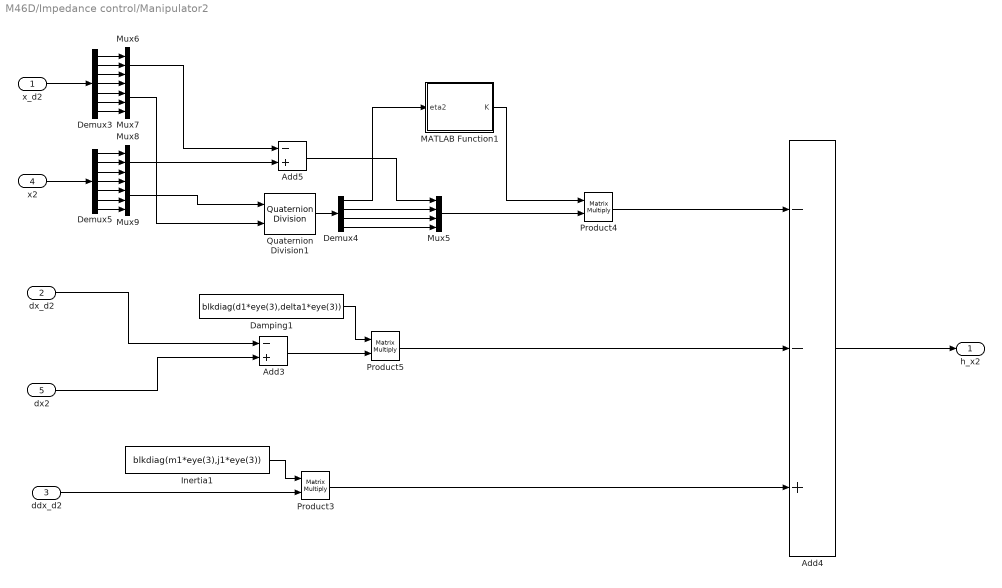
== system M46D/Impedance control/Manipulator2 ==
  x_d2 : Inport
  dx_d2 : Inport  Port=2
  ddx_d2 : Inport  Port=3
  x2 : Inport  Port=4
  dx2 : Inport  Port=5
  Add3 : Sum  Inputs=-+
  Add4 : Sum  Inputs=--+
  Add5 : Sum  Inputs=-+
  Damping1 : Constant  Value=blkdiag(d1*eye(3),delta1*eye(3))
  Demux3 : Demux  Outputs=7
  Demux4 : Demux
  Demux5 : Demux  Outputs=7
  Inertia1 : Constant  Value=blkdiag(m1*eye(3),j1*eye(3))
  MATLAB Function1 : MATLAB Function  TreatAsAtomicUnit=on
  Mux5 : Mux
  Mux6 : Mux  Inputs=3
  Mux7 : Mux
  Mux8 : Mux  Inputs=3
  Mux9 : Mux
  Product3 : Product  Multiplication=Matrix(*)
  Product4 : Product  Multiplication=Matrix(*)
  Product5 : Product  Multiplication=Matrix(*)
  Quaternion Division1 : aerolibutil/Quaternion Division
  h_x2 : Outport
  wires:
  Add3/1 -> Product5/2
  Damping1/1 -> Product5/1
  dx_d2/1 -> Add3/1
  dx2/1 -> Add3/2
  MATLAB Function1/1(K) -> Product4/1
  Demux4/1 -> MATLAB Function1/1(eta2)
  Add5/1 -> Mux5/1
  Demux4/2 -> Mux5/2
  Demux4/3 -> Mux5/3
  Demux4/4 -> Mux5/4
  x2/1 -> Demux5/1
  x_d2/1 -> Demux3/1
  Demux3/2 -> Mux6/2
  Demux3/1 -> Mux6/1
  Demux3/3 -> Mux6/3
  Demux3/4 -> Mux7/1
  Demux3/5 -> Mux7/2
  Demux3/6 -> Mux7/3
  Demux3/7 -> Mux7/4
  Demux5/2 -> Mux8/2
  Demux5/1 -> Mux8/1
  Demux5/3 -> Mux8/3
  Demux5/4 -> Mux9/1
  Demux5/5 -> Mux9/2
  Demux5/6 -> Mux9/3
  Demux5/7 -> Mux9/4
  Mux6/1 -> Add5/1
  Mux8/1 -> Add5/2
  Quaternion Division1/1 -> Demux4/1
  Mux9/1 -> Quaternion Division1/1
  Mux7/1 -> Quaternion Division1/2
  Mux5/1 -> Product4/2
  Inertia1/1 -> Product3/1
  ddx_d2/1 -> Product3/2
  Add4/1 -> h_x2/1
  Product4/1 -> Add4/1
  Product5/1 -> Add4/2
  Product3/1 -> Add4/3

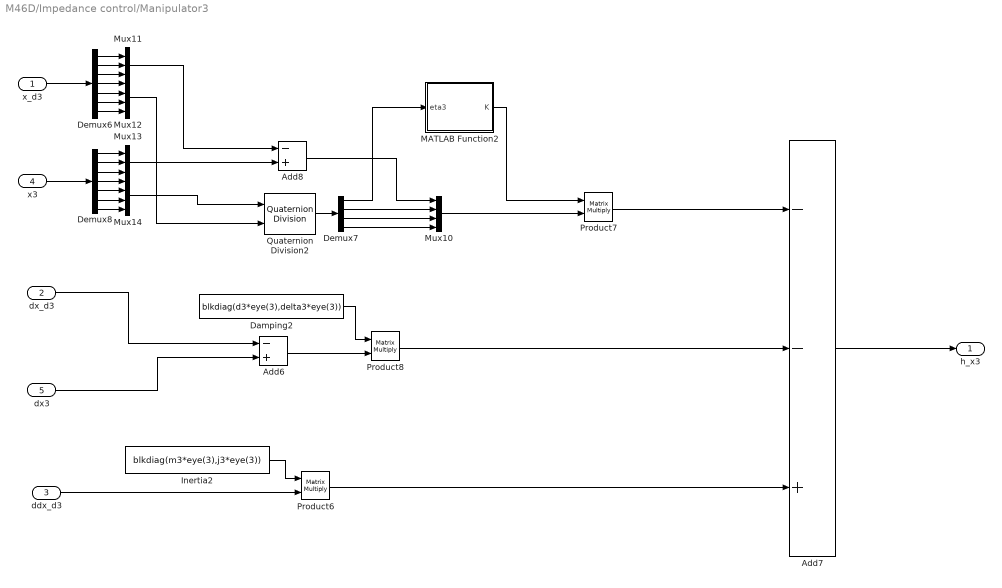
== system M46D/Impedance control/Manipulator3 ==
  x_d3 : Inport
  dx_d3 : Inport  Port=2
  ddx_d3 : Inport  Port=3
  x3 : Inport  Port=4
  dx3 : Inport  Port=5
  Add6 : Sum  Inputs=-+
  Add7 : Sum  Inputs=--+
  Add8 : Sum  Inputs=-+
  Damping2 : Constant  Value=blkdiag(d3*eye(3),delta3*eye(3))
  Demux6 : Demux  Outputs=7
  Demux7 : Demux
  Demux8 : Demux  Outputs=7
  Inertia2 : Constant  Value=blkdiag(m3*eye(3),j3*eye(3))
  MATLAB Function2 : MATLAB Function  TreatAsAtomicUnit=on
  Mux10 : Mux
  Mux11 : Mux  Inputs=3
  Mux12 : Mux
  Mux13 : Mux  Inputs=3
  Mux14 : Mux
  Product6 : Product  Multiplication=Matrix(*)
  Product7 : Product  Multiplication=Matrix(*)
  Product8 : Product  Multiplication=Matrix(*)
  Quaternion Division2 : aerolibutil/Quaternion Division
  h_x3 : Outport
  wires:
  Add6/1 -> Product8/2
  Damping2/1 -> Product8/1
  dx_d3/1 -> Add6/1
  dx3/1 -> Add6/2
  MATLAB Function2/1(K) -> Product7/1
  Demux7/1 -> MATLAB Function2/1(eta3)
  Add8/1 -> Mux10/1
  Demux7/2 -> Mux10/2
  Demux7/3 -> Mux10/3
  Demux7/4 -> Mux10/4
  x3/1 -> Demux8/1
  x_d3/1 -> Demux6/1
  Demux6/2 -> Mux11/2
  Demux6/1 -> Mux11/1
  Demux6/3 -> Mux11/3
  Demux6/4 -> Mux12/1
  Demux6/5 -> Mux12/2
  Demux6/6 -> Mux12/3
  Demux6/7 -> Mux12/4
  Demux8/2 -> Mux13/2
  Demux8/1 -> Mux13/1
  Demux8/3 -> Mux13/3
  Demux8/4 -> Mux14/1
  Demux8/5 -> Mux14/2
  Demux8/6 -> Mux14/3
  Demux8/7 -> Mux14/4
  Mux11/1 -> Add8/1
  Mux13/1 -> Add8/2
  Quaternion Division2/1 -> Demux7/1
  Mux14/1 -> Quaternion Division2/1
  Mux12/1 -> Quaternion Division2/2
  Mux10/1 -> Product7/2
  Inertia2/1 -> Product6/1
  ddx_d3/1 -> Product6/2
  Add7/1 -> h_x3/1
  Product7/1 -> Add7/1
  Product8/1 -> Add7/2
  Product6/1 -> Add7/3

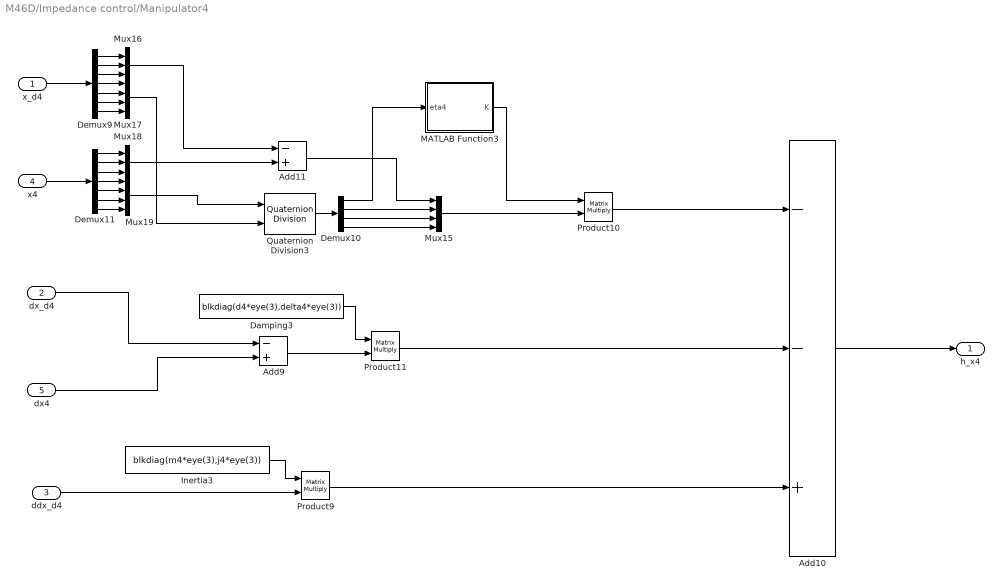
== system M46D/Impedance control/Manipulator4 ==
  x_d4 : Inport
  dx_d4 : Inport  Port=2
  ddx_d4 : Inport  Port=3
  x4 : Inport  Port=4
  dx4 : Inport  Port=5
  Add10 : Sum  Inputs=--+
  Add11 : Sum  Inputs=-+
  Add9 : Sum  Inputs=-+
  Damping3 : Constant  Value=blkdiag(d4*eye(3),delta4*eye(3))
  Demux10 : Demux
  Demux11 : Demux  Outputs=7
  Demux9 : Demux  Outputs=7
  Inertia3 : Constant  Value=blkdiag(m4*eye(3),j4*eye(3))
  MATLAB Function3 : MATLAB Function  TreatAsAtomicUnit=on
  Mux15 : Mux
  Mux16 : Mux  Inputs=3
  Mux17 : Mux
  Mux18 : Mux  Inputs=3
  Mux19 : Mux
  Product10 : Product  Multiplication=Matrix(*)
  Product11 : Product  Multiplication=Matrix(*)
  Product9 : Product  Multiplication=Matrix(*)
  Quaternion Division3 : aerolibutil/Quaternion Division
  h_x4 : Outport
  wires:
  Add9/1 -> Product11/2
  Damping3/1 -> Product11/1
  dx_d4/1 -> Add9/1
  dx4/1 -> Add9/2
  MATLAB Function3/1(K) -> Product10/1
  Demux10/1 -> MATLAB Function3/1(eta4)
  Add11/1 -> Mux15/1
  Demux10/2 -> Mux15/2
  Demux10/3 -> Mux15/3
  Demux10/4 -> Mux15/4
  x4/1 -> Demux11/1
  x_d4/1 -> Demux9/1
  Demux9/2 -> Mux16/2
  Demux9/1 -> Mux16/1
  Demux9/3 -> Mux16/3
  Demux9/4 -> Mux17/1
  Demux9/5 -> Mux17/2
  Demux9/6 -> Mux17/3
  Demux9/7 -> Mux17/4
  Demux11/2 -> Mux18/2
  Demux11/1 -> Mux18/1
  Demux11/3 -> Mux18/3
  Demux11/4 -> Mux19/1
  Demux11/5 -> Mux19/2
  Demux11/6 -> Mux19/3
  Demux11/7 -> Mux19/4
  Mux16/1 -> Add11/1
  Mux18/1 -> Add11/2
  Quaternion Division3/1 -> Demux10/1
  Mux19/1 -> Quaternion Division3/1
  Mux17/1 -> Quaternion Division3/2
  Mux15/1 -> Product10/2
  Inertia3/1 -> Product9/1
  ddx_d4/1 -> Product9/2
  Add10/1 -> h_x4/1
  Product10/1 -> Add10/1
  Product11/1 -> Add10/2
  Product9/1 -> Add10/3

== system M46D/Manipulator motion/AngVelo2Quat ==
  omega_o : Inport
  Constant : Constant  Value=0
  Gain : Gain  Gain=0.5
  Integrator : Integrator  InitialCondition=[1; 0; 0; 0]
  Mux : Mux  Inputs=2
  Quaternion Multiplication : aerolibutil/Quaternion Multiplication
  Scope : Scope
      settings: ShowLegends=on  SaveName=ScopeData9
  q_o : Outport
  wires:
  omega_o/1 -> Gain/1
  Gain/1 -> Mux/2
  Constant/1 -> Mux/1
  Quaternion Multiplication/1 -> Integrator/1
  Integrator/1 -> Quaternion Multiplication/2, Scope/1, q_o/1
  Mux/1 -> Quaternion Multiplication/1

== system M46D/Trajectory Generation/AngVelo2Quat ==
  omega_do : Inport
  Constant : Constant  Value=0
  Gain : Gain  Gain=0.5
  Integrator : Integrator  InitialCondition=[1; 0; 0; 0]
  Mux : Mux  Inputs=2
  Quaternion Multiplication : aerolibutil/Quaternion Multiplication
  Scope : Scope
      settings: ShowLegends=on  SaveName=ScopeData9
  q_do : Outport
  wires:
  omega_do/1 -> Gain/1
  Gain/1 -> Mux/2
  Constant/1 -> Mux/1
  Quaternion Multiplication/1 -> Integrator/1
  Integrator/1 -> Quaternion Multiplication/2, Scope/1, q_do/1
  Mux/1 -> Quaternion Multiplication/1

== matlab function M46D/Force//motion control/Manipulator 2/MATLAB Function ==
  data: u input; K output; k2 parameter; kappa2 parameter
function K = stiffness(u,k2,kappa2)
K = blkdiag(k2*eye(3),2*u*kappa2*eye(3));

== matlab function M46D/Force//motion control/Manipulator 1/MATLAB Function ==
  data: u input; K output; k1 parameter; kappa1 parameter
function K = stiffness(u,k1,kappa1)
K = blkdiag(k1*eye(3),2*u*kappa1*eye(3));

== matlab function M46D/Interaction Dynamics/MATLAB Function ==
  data: dx input; b output; r parameter
function b = constraintvector(dx,r)
b = [(dx(4:6)'*r(1:3))*dx(4:6)-(dx(4:6)'*dx(4:6))*r(1:3);
    zeros(3,1);
    (dx(4:6)'*r(4:6))*dx(4:6)-(dx(4:6)'*dx(4:6))*r(4:6);
    zeros(3,1)
    (dx(4:6)'*r(7:9))*dx(4:6)-(dx(4:6)'*dx(4:6))*r(7:9);
    zeros(3,1)
    (dx(4:6)'*r(10:12))*dx(4:6)-(dx(4:6)'*dx(4:6))*r(10:12);
    zeros(3,1)];

== matlab function M46D/Manipulator coordination/MATLAB Function3 ==
  data: r parameter; G output
function G = GraspMatrix(r)
G = [eye(3) zeros(3) eye(3) zeros(3) eye(3) zeros(3) eye(3) zeros(3);
    skew_sm(r(1:3)) eye(3) skew_sm(r(4:6)) eye(3) skew_sm(r(7:9)) eye(3) skew_sm(r(10:12)) eye(3)];

== matlab function M46D/Interaction Dynamics/MATLAB Function1 ==
  data: r parameter; A output
function A = constraintMatrix(r)
A = [-eye(3),skew_sm(r(1:3)),eye(3),zeros(3,21);
    zeros(3),-eye(3),zeros(3),eye(3),zeros(3,18);
    -eye(3),skew_sm(r(4:6)),zeros(3,6),eye(3),zeros(3,15);
    zeros(3),-eye(3),zeros(3,9),eye(3),zeros(3,12);
    -eye(3),skew_sm(r(7:9)),zeros(3,12),eye(3),zeros(3,9);
    zeros(3),-eye(3),zeros(3,15),eye(3),zeros(3,6);
    -eye(3),skew_sm(r(10:12)),zeros(3,18),eye(3),zeros(3);
    zeros(3),-eye(3),zeros(3,21),eye(3)];

== matlab function M46D/Manipulator coordination/MATLAB Function1 ==
  data: r parameter; G_Mplus output; m0 parameter; m1 parameter; m2 parameter; j0 parameter; j1 parameter; j2 parameter
function G_Mplus = geninvGraspM(r,m0,m1,m2,j0,j1,j2)
G_Mplus = [m1/m0*eye(3) (m1/j0*skew_sm(r(1:3)))';
    zeros(3) j1/j0*eye(3);
    m2/m0*eye(3) (m2/j0*skew_sm(r(4:6)))';
    zeros(3) j2/j0*eye(3)];

== matlab function M46D/Interaction Dynamics/MATLAB Function2 ==
  data: dx input; rot output; r parameter
function rot = framerotation(dx,r)
rot = [zeros(6,1);
    (dx(4:6)'*r(1:3))*dx(4:6)-(dx(4:6)'*dx(4:6))*r(1:3);
    zeros(3,1);
    (dx(4:6)'*r(4:6))*dx(4:6)-(dx(4:6)'*dx(4:6))*r(4:6);
    zeros(3,1);
    (dx(4:6)'*r(7:9))*dx(4:6)-(dx(4:6)'*dx(4:6))*r(7:9);
    zeros(3,1);
    (dx(4:6)'*r(10:12))*dx(4:6)-(dx(4:6)'*dx(4:6))*r(10:12);
    zeros(3,1)];

== matlab function M46D/Interaction Dynamics/MATLAB Function3 ==
  data: dx input; Cf output; j0 parameter
function Cf = CoriolisF(dx,j0)
Cf = [zeros(3,1);
      j0*skew_sm(dx(4:6))*dx(4:6)];

== matlab function M46D/Force//motion control/Manipulator 3/MATLAB Function ==
  data: u input; K output; k3 parameter; kappa3 parameter
function K = stiffness(u,k3,kappa3)
K = blkdiag(k3*eye(3),2*u*kappa3*eye(3));

== matlab function M46D/Interaction Dynamics/MATLAB Function4 ==
  data: dx input; rot output; r parameter
function rot = framerotation(dx,r)
rot = [zeros(6,1);
    skew_sm(dx(4:6))*r(1:3);
    zeros(3,1);
    skew_sm(dx(4:6))*r(4:6);
    zeros(3,1);
    skew_sm(dx(4:6))*r(7:9);
    zeros(3,1);
    skew_sm(dx(4:6))*r(10:12);
    zeros(3,1)];

== matlab function M46D/Force//motion control/Manipulator 2/MATLAB Function4 ==
  data: dx input; rot output; r parameter
function rot = framerotation(dx,r)
rot = [skew_sm(dx(4:6))*r(4:6);
    zeros(3,1)];

== matlab function M46D/Force//motion control/Manipulator 1/MATLAB Function4 ==
  data: dx input; rot output; r parameter
function rot = framerotation(dx,r)
rot = [skew_sm(dx(4:6))*r(1:3);
    zeros(3,1)];

== matlab function M46D/Force//motion control/Manipulator 1/MATLAB Function2 ==
  data: dx_d input; rot output; r parameter
function rot = framerotation(dx_d,r)
rot = [(dx_d(4:6)'*r(1:3))*dx_d(4:6)-(dx_d(4:6)'*dx_d(4:6))*r(1:3);
    zeros(3,1)];

== matlab function M46D/Force//motion control/Manipulator 2/MATLAB Function2 ==
  data: dx_d input; rot output; r parameter
function rot = framerotation(dx_d,r)
rot = [(dx_d(4:6)'*r(4:6))*dx_d(4:6)-(dx_d(4:6)'*dx_d(4:6))*r(4:6);
    zeros(3,1)];

== matlab function M46D/Interaction Dynamics/MATLAB Function5 ==
  data: x input; A_xyz output
function A_xyz = rotationMatrix(x)
A_xyz = [cos(x(5))*cos(x(6)) cos(x(4))*sin(x(6))+sin(x(4))*sin(x(5))*cos(x(6)) sin(x(4))*sin(x(6))-cos(x(4))*sin(x(5))*cos(x(6));
         -cos(x(5))*sin(x(6)) cos(x(4))*cos(x(6))-sin(x(4))*sin(x(5))*sin(x(6)) sin(x(4))*cos(x(6))+cos(x(4))*sin(x(5))*sin(x(6));
         -sin(x(4)) -sin(x(4))*cos(x(5)) cos(x(4))*cos(x(5))];

== matlab function M46D/Force//motion control/Manipulator 3/MATLAB Function2 ==
  data: dx_d input; rot output; r parameter
function rot = framerotation(dx_d,r)
rot = [(dx_d(4:6)'*r(7:9))*dx_d(4:6)-(dx_d(4:6)'*dx_d(4:6))*r(7:9);
    zeros(3,1)];

== matlab function M46D/Force//motion control/Manipulator 3/MATLAB Function4 ==
  data: dx input; rot output; r parameter
function rot = framerotation(dx,r)
rot = [skew_sm(dx(4:6))*r(7:9);
    zeros(3,1)];

== matlab function M46D/Force//motion control/Manipulator 4/MATLAB Function ==
  data: u input; K output; k4 parameter; kappa4 parameter
function K = stiffness(u,k4,kappa4)
K = blkdiag(k4*eye(3),2*u*kappa4*eye(3));

== matlab function M46D/Force//motion control/Manipulator 4/MATLAB Function2 ==
  data: dx_d input; rot output; r parameter
function rot = framerotation(dx_d,r)
rot = [(dx_d(4:6)'*r(10:12))*dx_d(4:6)-(dx_d(4:6)'*dx_d(4:6))*r(10:12);
    zeros(3,1)];

== matlab function M46D/Force//motion control/Manipulator 4/MATLAB Function4 ==
  data: dx input; rot output; r parameter
function rot = framerotation(dx,r)
rot = [skew_sm(dx(4:6))*r(10:12);
    zeros(3,1)];

== matlab function M46D/Kinematic Coordination/MATLAB Function3 ==
  data: r parameter; G output
function G = GraspMatrix(r)
G = [eye(3) zeros(3) eye(3) zeros(3) eye(3) zeros(3) eye(3) zeros(3);
    skew_sm(r(1:3)) eye(3) skew_sm(r(4:6)) eye(3) skew_sm(r(7:9)) eye(3) skew_sm(r(10:12)) eye(3)];

== matlab function M46D/Kinematic Coordination/MATLAB Function ==
  data: p_do input; q_do input; x_d output; r parameter
function x_d = manipulatorpose(p_do,q_do,r)
pq_d1 = quatmultiply(quatconj(q_do'),quatmultiply([0 r(1:3)'],q_do'))';
pq_d2 = quatmultiply(quatconj(q_do'),quatmultiply([0 r(4:6)'],q_do'))';
pq_d3 = quatmultiply(quatconj(q_do'),quatmultiply([0 r(7:9)'],q_do'))';
pq_d4 = quatmultiply(quatconj(q_do'),quatmultiply([0 r(10:12)'],q_do'))';


x_d = [p_do + pq_d1(2:4);
        q_do;
        p_do + pq_d2(2:4);
        q_do;
        p_do + pq_d3(2:4);
        q_do;
        p_do + pq_d4(2:4);
        q_do ];

== matlab function M46D/Kinematic Coordination/MATLAB Function1 ==
  data: dx_do input; b output; r parameter
function b = centripetalforce(dx_do,r)
b = [skew_sm(dx_do(4:6))*skew_sm(dx_do(4:6))*r(1:3);
    zeros(3,1);
    skew_sm(dx_do(4:6))*skew_sm(dx_do(4:6))*r(4:6);
    zeros(3,1);
    skew_sm(dx_do(4:6))*skew_sm(dx_do(4:6))*r(7:9);
    zeros(3,1);
    skew_sm(dx_do(4:6))*skew_sm(dx_do(4:6))*r(10:12)
    zeros(3,1)];

== matlab function M46D/Inverse Dynamics/MATLAB Function ==
  data: dx_do input; C_o output; j0 parameter
function C_o = Coriolis(dx_do,j0)
C_o = [zeros(3,6);
        zeros(3) j0*skew_sm(dx_do(4:6))];

== matlab function M46D/Inverse Dynamics/MATLAB Function3 ==
  data: r parameter; G output
function G = GraspMatrix(r)
G = [eye(3) zeros(3) eye(3) zeros(3) eye(3) zeros(3) eye(3) zeros(3);
    skew_sm(r(1:3)) eye(3) skew_sm(r(4:6)) eye(3) skew_sm(r(7:9)) eye(3) skew_sm(r(10:12)) eye(3)];

== matlab function M46D/Impedance control/Manipulator1/MATLAB Function ==
  data: eta1 input; K output; k1 parameter; kappa1 parameter
function K = stiffness(eta1,k1,kappa1)
K = blkdiag(k1*eye(3),2*eta1*kappa1*eye(3));

== matlab function M46D/Impedance control/Manipulator2/MATLAB Function1 ==
  data: eta2 input; K output; k2 parameter; kappa2 parameter
function K = stiffness(eta2,k2,kappa2)
K = blkdiag(k2*eye(3),2*eta2*kappa2*eye(3));

== matlab function M46D/Impedance control/Manipulator3/MATLAB Function2 ==
  data: eta3 input; K output; k3 parameter; kappa3 parameter
function K = stiffness(eta3,k3,kappa3)
K = blkdiag(k3*eye(3),2*eta3*kappa3*eye(3));

== matlab function M46D/Impedance control/Manipulator4/MATLAB Function3 ==
  data: eta4 input; K output; k4 parameter; kappa4 parameter
function K = stiffness(eta4,k4,kappa4)
K = blkdiag(k4*eye(3),2*eta4*kappa4*eye(3));

== matlab function M46D/Manipulator dynamics/MATLAB Function ==
  data: r parameter; Ared output
function Ared = ReducedConstraintMAtrix(r)
Ared = [-eye(3) skew_sm(r(4:6)-r(1:3)) eye(3) zeros(3,15);
        zeros(3) -eye(3) zeros(3) eye(3) zeros(3,12);
        -eye(3) skew_sm(r(7:9)-r(1:3)) zeros(3,6) eye(3) zeros(3,9);
        zeros(3) -eye(3) zeros(3,9) eye(3) zeros(3,6);
        -eye(3) skew_sm(r(10:12)-r(1:3)) zeros(3,12) eye(3) zeros(3);
        zeros(3) -eye(3) zeros(3,15) eye(3)];

== matlab function M46D/Manipulator dynamics/MATLAB Function1 ==
  data: r parameter; bred output; dx input
function bred = ReducedCentripetalvector(r,dx)
bred = [skew_sm(dx(4:6))*skew_sm(dx(4:6))*(r(4:6)-r(1:3));
    zeros(3,1);
    skew_sm(dx(4:6))*skew_sm(dx(4:6))*(r(7:9)-r(1:3));
    zeros(3,1);
    skew_sm(dx(4:6))*skew_sm(dx(4:6))*(r(10:12)-r(1:3));
    zeros(3,1)];

== matlab function M46D/Interaction dynamics/MATLAB Function ==
  data: G input; Mapp output; M input; m0 parameter; j0 parameter
function Mapp = ApparentInertia(G,M,m0,j0)
Mapp = blkdiag(m0*eye(3),j0*eye(3)) + G*M*G';

== matlab function M46D/Interaction dynamics/MATLAB Function3 ==
  data: r parameter; G output
function G = GraspMatrix(r)
G = [eye(3) zeros(3) eye(3) zeros(3) eye(3) zeros(3) eye(3) zeros(3);
    skew_sm(r(1:3)) eye(3) skew_sm(r(4:6)) eye(3) skew_sm(r(7:9)) eye(3) skew_sm(r(10:12)) eye(3)];

== matlab function M46D/Interaction dynamics/MATLAB Function1 ==
  data: dx input; hcoriolis output; j0 parameter
function hcoriolis = CoriolisForce(dx,j0)
hcoriolis = [zeros(3,1);
        j0*skew_sm(dx(4:6))*dx(4:6)];

== matlab function M46D/Interaction dynamics/MATLAB Function2 ==
  data: dx input; b output; r parameter
function b = centripetalforce(dx,r)
b = [skew_sm(dx(4:6))*skew_sm(dx(4:6))*r(1:3);
    zeros(3,1);
    skew_sm(dx(4:6))*skew_sm(dx(4:6))*r(4:6);
    zeros(3,1);
    skew_sm(dx(4:6))*skew_sm(dx(4:6))*r(7:9);
    zeros(3,1);
    skew_sm(dx(4:6))*skew_sm(dx(4:6))*r(10:12)
    zeros(3,1)];

== matlab function M46D/Manipulator motion/MATLAB Function3 ==
  data: r parameter; G output
function G = GraspMatrix(r)
G = [eye(3) zeros(3) eye(3) zeros(3) eye(3) zeros(3) eye(3) zeros(3);
    skew_sm(r(1:3)) eye(3) skew_sm(r(4:6)) eye(3) skew_sm(r(7:9)) eye(3) skew_sm(r(10:12)) eye(3)];

== matlab function M46D/Manipulator motion/MATLAB Function ==
  data: p_o input; q_o input; x output; r parameter
function x = manipulatorpose(p_o,q_o,r)
pq1 = quatmultiply(quatconj(q_o'),quatmultiply([0 r(1:3)'],q_o'))';
pq2 = quatmultiply(quatconj(q_o'),quatmultiply([0 r(4:6)'],q_o'))';
pq3 = quatmultiply(quatconj(q_o'),quatmultiply([0 r(7:9)'],q_o'))';
pq4 = quatmultiply(quatconj(q_o'),quatmultiply([0 r(10:12)'],q_o'))';


x = [p_o + pq1(2:4);
        q_o;
        p_o + pq2(2:4);
        q_o;
        p_o + pq3(2:4);
        q_o;
        p_o + pq4(2:4);
        q_o ];

== matlab function M46D/Nullspace/MATLAB Function ==
  data: r parameter; Ared output
function Ared = ReducedConstraintMAtrix(r)
Ared = [-eye(3) skew_sm(r(4:6)-r(1:3)) eye(3) zeros(3,15);
        zeros(3) -eye(3) zeros(3) eye(3) zeros(3,12);
        -eye(3) skew_sm(r(7:9)-r(1:3)) zeros(3,6) eye(3) zeros(3,9);
        zeros(3) -eye(3) zeros(3,9) eye(3) zeros(3,6);
        -eye(3) skew_sm(r(10:12)-r(1:3)) zeros(3,12) eye(3) zeros(3);
        zeros(3) -eye(3) zeros(3,15) eye(3)];

== matlab function M46D/Allocator/MATLAB Function1 ==
  data: r parameter; bred output; dx input
function bred = ReducedCentripetalvector(r,dx)
bred = [skew_sm(dx(4:6))*skew_sm(dx(4:6))*(r(4:6)-r(1:3));
    zeros(3,1);
    skew_sm(dx(4:6))*skew_sm(dx(4:6))*(r(7:9)-r(1:3));
    zeros(3,1);
    skew_sm(dx(4:6))*skew_sm(dx(4:6))*(r(10:12)-r(1:3));
    zeros(3,1)];

== matlab function M46D/Allocator/MATLAB Function ==
  data: r parameter; Ared output
function Ared = ReducedConstraintMAtrix(r)
Ared = [-eye(3) skew_sm(r(4:6)-r(1:3)) eye(3) zeros(3,15);
        zeros(3) -eye(3) zeros(3) eye(3) zeros(3,12);
        -eye(3) skew_sm(r(7:9)-r(1:3)) zeros(3,6) eye(3) zeros(3,9);
        zeros(3) -eye(3) zeros(3,9) eye(3) zeros(3,6);
        -eye(3) skew_sm(r(10:12)-r(1:3)) zeros(3,12) eye(3) zeros(3);
        zeros(3) -eye(3) zeros(3,15) eye(3)];
